simulink model "bp7a_model"  (R2019b)
settings: Solver=ode15s  StartTime=0.0  StopTime=10.0  RelTol=1e-10
PreLoadFcn:
  | ww=[1e-5,1e5]; N=27; a=0; b=0;
libraries: cstblocks x5
settings Model: Creator=Professor Dingyu Xue  LastModifiedBy=xuedi
settings DataIOCC: SaveFormat=Array  ReturnWorkspaceOutputs=off
settings DebuggingCC: AlgebraicLoopMsg=none  ArithmeticOperatorsInVariantConditions=warning
settings SFSimCC: SimUseLocalCustomCode=off  CustomCodeUndefinedFunction=UseInterfaceOnly
settings RTWCC: RTWUseLocalCustomCode=off
settings CodeAppCC: StateflowObjectComments=on

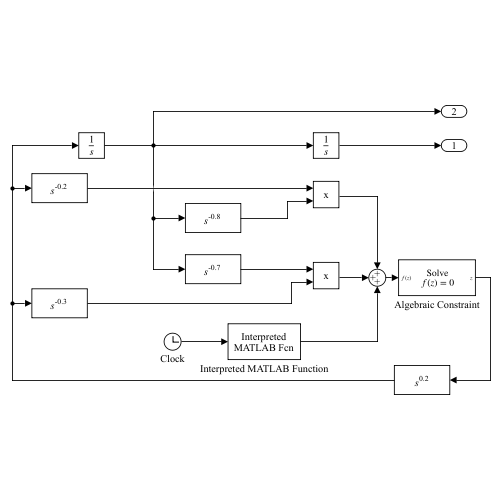
[thumbnail: Simulink's stored preview of the top-level diagram]
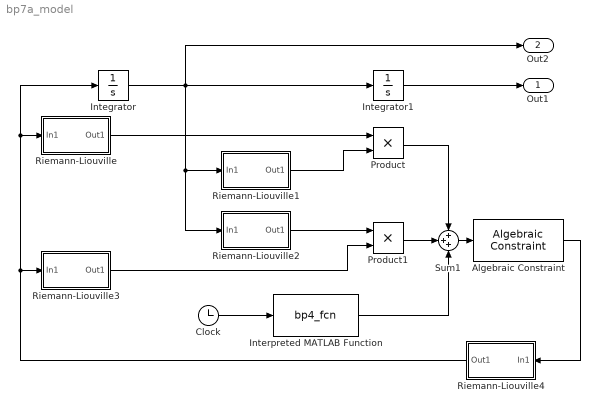
== system bp7a_model ==
  Algebraic Constraint : AlgebraicConstraint
  Clock : Clock
  Integrator : Integrator  InitialCondition=a
  Integrator1 : Integrator  InitialCondition=b
  Interpreted MATLAB Function : MATLABFcn  MATLABFcn=bp4_fcn
  Product : Product
  Product1 : Product
  Riemann-Liouville : Subsystem  mask{gam=-0.2, ww=ww, n=N, kF1=off, kF=Oustaloup filter}
      mask prompts: gam "Derivative order gamma"; ww "Frequency range [wb,wh]"; n "Apprixmation order"; kF1 "Is a low-pass filter required?"; kF "Filter type"
      mask init:
      | wb=ww(1); wh=ww(2); 
      |    if isnumeric(gam), str=['{\its}^{' num2str(gam) '}']; 
      |    else, str='{\its}^{\gamma}'; end
      |    switch kF
      |       case 1, G=ousta_fod(gam,n,wb,wh);
      |       case 2, G=new_fod(gam,n,wb,wh); 
      |       case 3, G=matsuda_fod(gam,n,wb,wh); 
      |       case 4, G=srid_fod(gam,0.01,n);
      |    end
      |    T=1e-6/wh; if kF1==1, G=G*tf(1,[T 1]); end
      mask TypeOptions kF: Oustaloup filter | Modified Oustaloup filter | Matsuda-Fujii filter | Discrete step invariant filter
      mask Display: disp(str,'texmode','on')
  Riemann-Liouville1 : Subsystem  mask{gam=-0.8, ww=ww, n=N, kF1=off, kF=Oustaloup filter}
      mask prompts: gam "Derivative order gamma"; ww "Frequency range [wb,wh]"; n "Apprixmation order"; kF1 "Is a low-pass filter required?"; kF "Filter type"
      mask init: same as bp7a_model/Riemann-Liouville
      mask TypeOptions kF: Oustaloup filter | Modified Oustaloup filter | Matsuda-Fujii filter | Discrete step invariant filter
      mask Display: disp(str,'texmode','on')
  Riemann-Liouville2 : Subsystem  mask{gam=-0.7, ww=ww, n=N, kF1=off, kF=Oustaloup filter}
      mask prompts: gam "Derivative order gamma"; ww "Frequency range [wb,wh]"; n "Apprixmation order"; kF1 "Is a low-pass filter required?"; kF "Filter type"
      mask init: same as bp7a_model/Riemann-Liouville
      mask TypeOptions kF: Oustaloup filter | Modified Oustaloup filter | Matsuda-Fujii filter | Discrete step invariant filter
      mask Display: disp(str,'texmode','on')
  Riemann-Liouville3 : Subsystem  mask{gam=-0.3, ww=ww, n=N, kF1=off, kF=Oustaloup filter}
      mask prompts: gam "Derivative order gamma"; ww "Frequency range [wb,wh]"; n "Apprixmation order"; kF1 "Is a low-pass filter required?"; kF "Filter type"
      mask init: same as bp7a_model/Riemann-Liouville
      mask TypeOptions kF: Oustaloup filter | Modified Oustaloup filter | Matsuda-Fujii filter | Discrete step invariant filter
      mask Display: disp(str,'texmode','on')
  Riemann-Liouville4 : Subsystem  mask{gam=0.2, ww=ww, n=N, kF1=off, kF=Oustaloup filter}
      mask prompts: gam "Derivative order gamma"; ww "Frequency range [wb,wh]"; n "Apprixmation order"; kF1 "Is a low-pass filter required?"; kF "Filter type"
      mask init: same as bp7a_model/Riemann-Liouville
      mask TypeOptions kF: Oustaloup filter | Modified Oustaloup filter | Matsuda-Fujii filter | Discrete step invariant filter
      mask Display: disp(str,'texmode','on')
  Sum1 : Sum  Inputs=+++
  Out1 : Outport
  Out2 : Outport  Port=2
  wires:
  Clock/1 -> Interpreted MATLAB Function/1
  Product1/1 -> Sum1/2
  Product/1 -> Sum1/1
  Sum1/1 -> Algebraic Constraint/1
  Integrator1/1 -> Out1/1
  Interpreted MATLAB Function/1 -> Sum1/3
  Integrator/1 -> Out2/1, Integrator1/1, Riemann-Liouville2/1(In1), Riemann-Liouville1/1(In1)
  Algebraic Constraint/1 -> Riemann-Liouville4/1(In1)
  Riemann-Liouville/1(Out1) -> Product/1
  Riemann-Liouville1/1(Out1) -> Product/2
  Riemann-Liouville2/1(Out1) -> Product1/1
  Riemann-Liouville3/1(Out1) -> Product1/2
  Riemann-Liouville4/1(Out1) -> Riemann-Liouville3/1(In1), Integrator/1, Riemann-Liouville/1(In1)

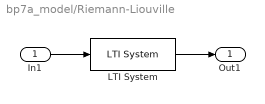
== system bp7a_model/Riemann-Liouville ==
  In1 : Inport
  LTI System : cstblocks/LTI System  sys=G  IC=[]
  Out1 : Outport
  wires:
  LTI System/1 -> Out1/1
  In1/1 -> LTI System/1

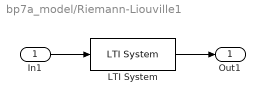
== system bp7a_model/Riemann-Liouville1 ==
  In1 : Inport
  LTI System : cstblocks/LTI System  sys=G  IC=[]
  Out1 : Outport
  wires:
  In1/1 -> LTI System/1
  LTI System/1 -> Out1/1

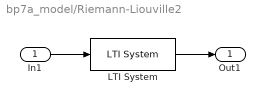
== system bp7a_model/Riemann-Liouville2 ==
  In1 : Inport
  LTI System : cstblocks/LTI System  sys=G  IC=[]
  Out1 : Outport
  wires:
  LTI System/1 -> Out1/1
  In1/1 -> LTI System/1

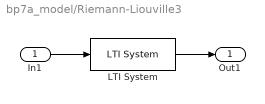
== system bp7a_model/Riemann-Liouville3 ==
  In1 : Inport
  LTI System : cstblocks/LTI System  sys=G  IC=[]
  Out1 : Outport
  wires:
  In1/1 -> LTI System/1
  LTI System/1 -> Out1/1

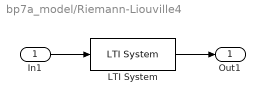
== system bp7a_model/Riemann-Liouville4 ==
  In1 : Inport
  LTI System : cstblocks/LTI System  sys=G  IC=[]
  Out1 : Outport
  wires:
  LTI System/1 -> Out1/1
  In1/1 -> LTI System/1
